simulink subsystem "mmc_fb_arm"  (R2026a)
settings: Solver=VariableStepAuto
settings Model: Creator=zheng  LastModifiedBy=zheng

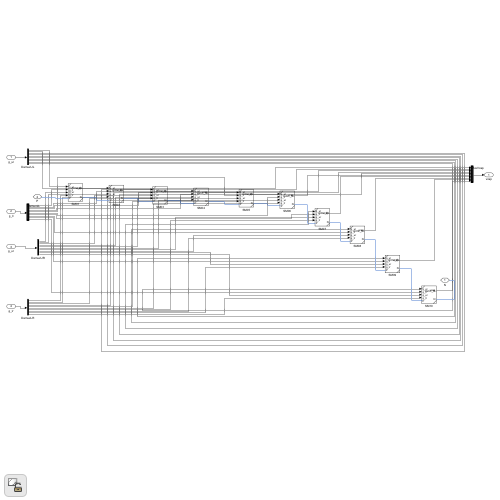
[thumbnail: Simulink's stored preview of the top-level diagram]
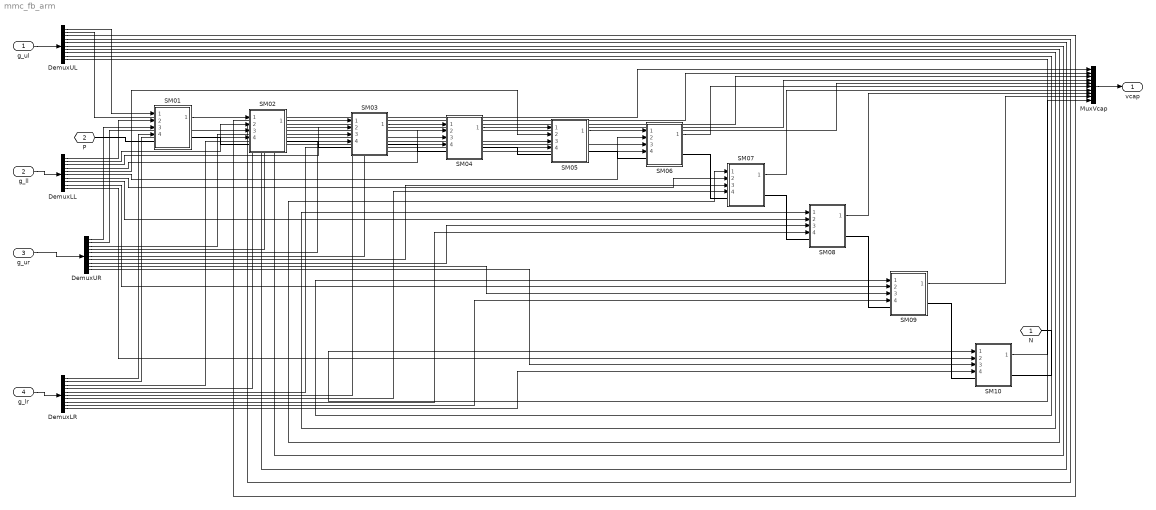
== system mmc_fb_arm ==
  g_ul : Inport
  g_ll : Inport  Port=2
  g_ur : Inport  Port=3
  g_lr : Inport  Port=4
  DemuxLL : Demux  Outputs=10
  DemuxLR : Demux  Outputs=10
  DemuxUL : Demux  Outputs=10
  DemuxUR : Demux  Outputs=10
  MuxVcap : Mux  Inputs=10
  SM01 : Subsystem  ReferencedSubsystem=mmc_fb_submodule
  SM02 : Subsystem  ReferencedSubsystem=mmc_fb_submodule
  SM03 : Subsystem  ReferencedSubsystem=mmc_fb_submodule
  SM04 : Subsystem  ReferencedSubsystem=mmc_fb_submodule
  SM05 : Subsystem  ReferencedSubsystem=mmc_fb_submodule
  SM06 : Subsystem  ReferencedSubsystem=mmc_fb_submodule
  SM07 : Subsystem  ReferencedSubsystem=mmc_fb_submodule
  SM08 : Subsystem  ReferencedSubsystem=mmc_fb_submodule
  SM09 : Subsystem  ReferencedSubsystem=mmc_fb_submodule
  SM10 : Subsystem  ReferencedSubsystem=mmc_fb_submodule
  N : PMIOPort  Side=Right  ConnectionType=Connection: foundation.electrical.electrical
  P : PMIOPort  Port=2  Side=Left  ConnectionType=Connection: foundation.electrical.electrical
  vcap : Outport
  wires:
  g_ul/1 -> DemuxUL/1
  g_ll/1 -> DemuxLL/1
  g_ur/1 -> DemuxUR/1
  g_lr/1 -> DemuxLR/1
  MuxVcap/1 -> vcap/1
  DemuxUL/1 -> SM01/1
  DemuxLL/1 -> SM01/2
  DemuxUR/1 -> SM01/3
  DemuxLR/1 -> SM01/4
  SM01/1 -> MuxVcap/1
  DemuxUL/2 -> SM02/1
  DemuxLL/2 -> SM02/2
  DemuxUR/2 -> SM02/3
  DemuxLR/2 -> SM02/4
  SM02/1 -> MuxVcap/2
  DemuxUL/3 -> SM03/1
  DemuxLL/3 -> SM03/2
  DemuxUR/3 -> SM03/3
  DemuxLR/3 -> SM03/4
  SM03/1 -> MuxVcap/3
  DemuxUL/4 -> SM04/1
  DemuxLL/4 -> SM04/2
  DemuxUR/4 -> SM04/3
  DemuxLR/4 -> SM04/4
  SM04/1 -> MuxVcap/4
  DemuxUL/5 -> SM05/1
  DemuxLL/5 -> SM05/2
  DemuxUR/5 -> SM05/3
  DemuxLR/5 -> SM05/4
  SM05/1 -> MuxVcap/5
  DemuxUL/6 -> SM06/1
  DemuxLL/6 -> SM06/2
  DemuxUR/6 -> SM06/3
  DemuxLR/6 -> SM06/4
  SM06/1 -> MuxVcap/6
  DemuxUL/7 -> SM07/1
  DemuxLL/7 -> SM07/2
  DemuxUR/7 -> SM07/3
  DemuxLR/7 -> SM07/4
  SM07/1 -> MuxVcap/7
  DemuxUL/8 -> SM08/1
  DemuxLL/8 -> SM08/2
  DemuxUR/8 -> SM08/3
  DemuxLR/8 -> SM08/4
  SM08/1 -> MuxVcap/8
  DemuxUL/9 -> SM09/1
  DemuxLL/9 -> SM09/2
  DemuxUR/9 -> SM09/3
  DemuxLR/9 -> SM09/4
  SM09/1 -> MuxVcap/9
  DemuxUL/10 -> SM10/1
  DemuxLL/10 -> SM10/2
  DemuxUR/10 -> SM10/3
  DemuxLR/10 -> SM10/4
  SM10/1 -> MuxVcap/10
  connections:
  P/RConn1 -- SM01/LConn1
  SM01/RConn1 -- SM02/LConn1
  SM02/RConn1 -- SM03/LConn1
  SM03/RConn1 -- SM04/LConn1
  SM04/RConn1 -- SM05/LConn1
  SM05/RConn1 -- SM06/LConn1
  SM06/RConn1 -- SM07/LConn1
  SM07/RConn1 -- SM08/LConn1
  SM08/RConn1 -- SM09/LConn1
  SM09/RConn1 -- SM10/LConn1
  SM10/RConn1 -- N/RConn1
